simulink model "diagrama"  (R2020a)
settings: Solver=VariableStepAuto  StartTime=0.0  StopTime=10.0  RelTol=1e-3
settings Model: Creator=Camil  LastModifiedBy=Camil

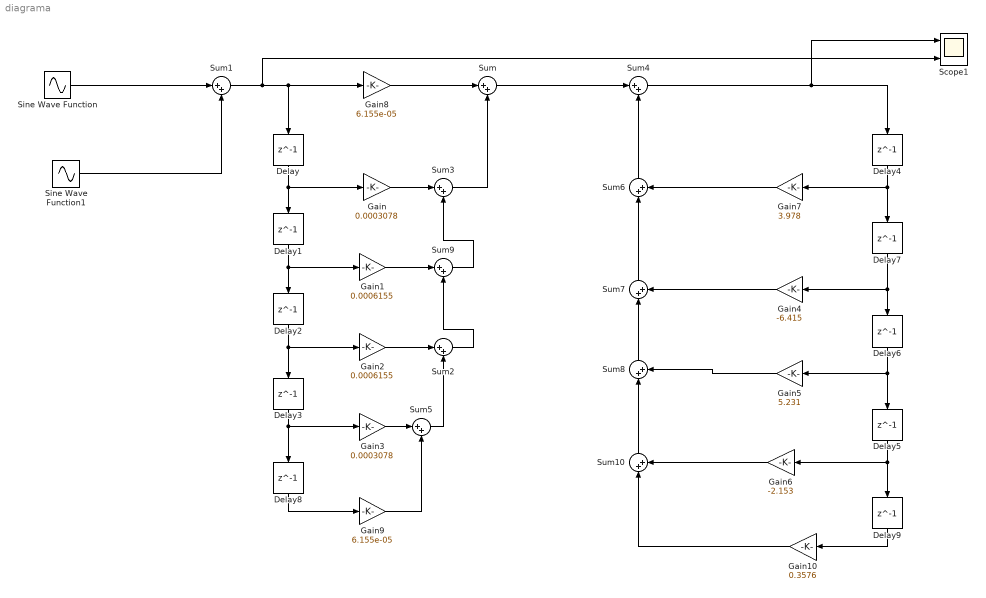
== system diagrama ==
  Delay{,1..9} (10 alike) : Delay  DelayLength=1  InitialCondition=0
  Gain : Gain  Gain=0.0003078
  Gain1 : Gain  Gain=0.0006155
  Gain10 : Gain  Gain=0.3576
  Gain2 : Gain  Gain=0.0006155
  Gain3 : Gain  Gain=0.0003078
  Gain4 : Gain  Gain=-6.415
  Gain5 : Gain  Gain=5.231
  Gain6 : Gain  Gain=-2.153
  Gain7 : Gain  Gain=3.978
  Gain8 : Gain  Gain=6.155e-05
  Gain9 : Gain  Gain=6.155e-05
  Scope1 : Scope  NumInputPorts=2
  Sine Wave Function : Sin  SineType=Sample based  Amplitude=2  Samples=5  SampleTime=0.001
  Sine Wave Function1 : Sin  SineType=Sample based  Samples=5  SampleTime=0.001
  Sum{,1..10} (11 alike) : Sum  Inputs=|++
  wires:
  Sine Wave Function/1 -> Sum1/1
  Sine Wave Function1/1 -> Sum1/2
  Sum1/1 -> Scope1/2, Gain8/1, Delay/1
  Delay1/1 -> Gain1/1, Delay2/1
  Delay/1 -> Gain/1, Delay1/1
  Delay2/1 -> Gain2/1, Delay3/1
  Gain/1 -> Sum3/1
  Gain1/1 -> Sum9/1
  Gain2/1 -> Sum2/1
  Sum2/1 -> Sum9/2
  Sum9/1 -> Sum3/2
  Sum3/1 -> Sum/2
  Sum/1 -> Sum4/1
  Sum4/1 -> Scope1/1, Delay4/1
  Delay4/1 -> Gain7/1, Delay7/1
  Delay7/1 -> Gain4/1, Delay6/1
  Delay6/1 -> Delay5/1, Gain5/1
  Gain7/1 -> Sum6/2
  Sum6/1 -> Sum4/2
  Sum7/1 -> Sum6/1
  Gain4/1 -> Sum7/2
  Sum8/1 -> Sum7/1
  Gain5/1 -> Sum8/2
  Gain8/1 -> Sum/1
  Sum5/1 -> Sum2/2
  Gain3/1 -> Sum5/1
  Delay8/1 -> Gain9/1
  Delay3/1 -> Delay8/1, Gain3/1
  Gain9/1 -> Sum5/2
  Delay9/1 -> Gain10/1
  Delay5/1 -> Delay9/1, Gain6/1
  Gain6/1 -> Sum10/2
  Sum10/1 -> Sum8/1
  Gain10/1 -> Sum10/1
